simulink model "nao_linear"  (R2025a)
settings: Solver=VariableStepAuto  StartTime=0.0  StopTime=50.0  RelTol=1e-3
values from neighbouring files (symbols this model uses):
  b = 0.010681    [equations_aeropendulum.m]
  den = [1, b/J, (m*g/J) * L1 * cos(theta)]    [equations_aeropendulum.m]
  g = 9.81    [equations_aeropendulum.m]
  J = 0.020218    [equations_aeropendulum.m]
  K = 0.000166    [equations_aeropendulum.m]
  L1 = 0.177    [equations_aeropendulum.m]
  L2 = 0.45    [equations_aeropendulum.m]
  m = 0.218    [equations_aeropendulum.m]
  num = [K * L2 * 2 * pwm / J]    [equations_aeropendulum.m]
  pwm = 89    [equations_aeropendulum.m]
  theta = 90    [equations_aeropendulum.m]
libraries: slpidlib x1
settings Model: Creator=edutera  LastModifiedBy=edutera

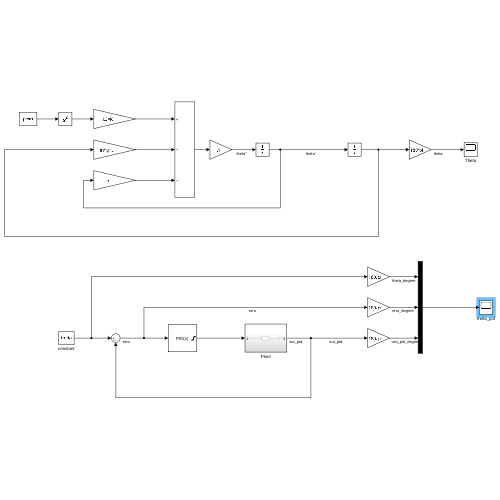
[thumbnail: Simulink's stored preview of the top-level diagram]
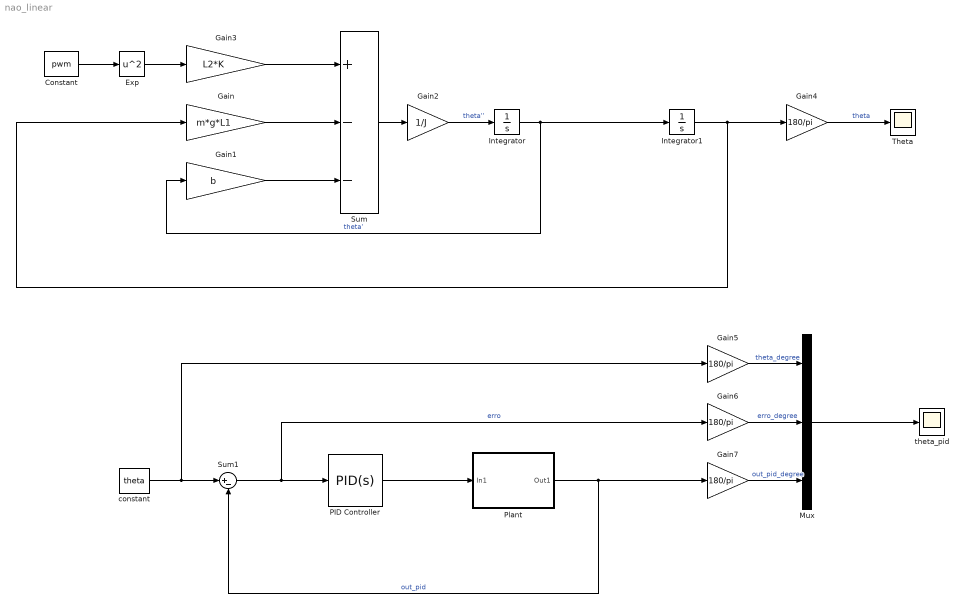
== system nao_linear ==
  Constant : Constant  Value=pwm
  Exp : Math  Operator=square
  Gain : Gain  Gain=m*g*L1
  Gain1 : Gain  Gain=b
  Gain2 : Gain  Gain=1/J
  Gain3 : Gain  Gain=L2*K
  Gain{4..7} (4 alike) : Gain  Gain=180/pi
  Integrator : Integrator
  Integrator1 : Integrator
  Mux : Mux  Inputs=3
  PID Controller : slpidlib/PID Controller  Controller=PID  Form=Parallel  TimeDomain=Continuous-time  UseExternalTs=off  SampleTime=-1  IntegratorMethod=Forward Euler  FilterMethod=Forward Euler  ControllerParametersSource=internal  P=0.5  I=0.06  UseKiTs=off  D=0.9  UseExternalDerivativeSource=off  N=100  UseFilter=on  TunerSelectOption=Transfer Function Based (PID Tuner App)  InitialConditionSource=internal  InitialConditionForIntegrator=0  InitialConditionForFilter=0  DifferentiatorICPrevScaledInput=0  ExternalReset=none  TrackingMode=off  Kt=1  LimitOutput=on  SatLimitsSource=internal  UpperSaturationLimit=255  LowerSaturationLimit=0  LinearizeAsGain=on  AntiWindupMode=clamping  Kb=1  LimitIntegrator=off  UpperIntegratorSaturationLimit=inf  LowerIntegratorSaturationLimit=-inf  POutMin=[]  POutMax=[]  IOutMin=[]  IOutMax=[]  DOutMin=[]  DOutMax=[]  NOutMin=[]  NOutMax=[]  SumOutMin=[]  SumOutMax=[]  SaturationOutMin=[]  SaturationOutMax=[]  PParamMin=[]  PParamMax=[]  IParamMin=[]  IParamMax=[]  DParamMin=[]  DParamMax=[]  NParamMin=[]  NParamMax=[]  KbParamMin=[]  KbParamMax=[]  KtParamMin=[]  KtParamMax=[]  KbOutMin=[]  KbOutMax=[]  KtOutMin=[]  KtOutMax=[]  IntegratorOutMin=[]  IntegratorOutMax=[]  FilterOutMin=[]  FilterOutMax=[]  SumI1OutMin=[]  SumI1OutMax=[]  SumI2OutMin=[]  SumI2OutMax=[]  SumI3OutMin=[]  SumI3OutMax=[]  SumI4OutMin=[]  SumI4OutMax=[]  SumDOutMin=[]  SumDOutMax=[]  DifferentiatorOutMin=[]  DifferentiatorOutMax=[]  FilterDiffOutCoefMin=[]  FilterDiffOutCoefMax=[]  ReciprocalOutMin=[]  ReciprocalOutMax=[]  SumDenOutMin=[]  SumDenOutMax=[]  SumNumOutMin=[]  SumNumOutMax=[]  DivideOutMin=[]  DivideOutMax=[]  UdiffTsProdOutMin=[]  UdiffTsProdOutMax=[]  NTsProdOutMin=[]  NTsProdOutMax=[]  UintegralTsProdOutMin=[]  UintegralTsProdOutMax=[]  UngainTsProdOutMin=[]  UngainTsProdOutMax=[]  ClampingZeroOutDataTypeStr=Inherit: Inherit via back propagation  ClampingZeroOutMin=[]  ClampingZeroOutMax=[]  FilterDenConstantOutDataTypeStr=Inherit: Inherit via back propagation  FilterDenConstantOutMin=[]  FilterDenConstantOutMax=[]  PCopyOutDataTypeStr=Inherit: Inherit via back propagation  PCopyOutMin=[]  PCopyOutMax=[]  NCopyOutDataTypeStr=Inherit: Inherit via back propagation  NCopyOutMin=[]  NCopyOutMax=[]  IntegratorContinuousStateAttributes=''  IntegratorStateMustResolveToSignalObject=off  IntegratorRTWStateStorageClass=Auto  FilterContinuousStateAttributes=''  FilterStateMustResolveToSignalObject=off  FilterRTWStateStorageClass=Auto  ParallelPVariant=InternalParameters  IdealPVariant=Disabled  IVariant=InternalParameters  DVariant=InternalParameters  IntegratorVariant=Continuous  SatVariant=Enabled  AWVariant=ContClampingParallel  PCopyVariant=Disabled  TRVariant=Disabled  FdbkBlocksVariant=Forward  IdealPFdbkVariant=Disabled  SatFdbkVariant=Disabled  DerivativeFilterVariant=ContFilter  NVariant=InternalParameters  NCopyVariant=Disabled  FilterICVariant=InternalICsFilter  IntegratorICVariant=InternalICs  ExternalResetVariant=Disabled  TRSumVariant=Passthrough  SumFdbkVariant=Disabled  SumVariant=Sum_PID  TsampFilterVariant=InternalTs  TsampNgainVariant=Passthrough  TsampIntegralVariant=Disabled_SignalSpec  ExternalSaturationOutDataTypeStr=Inherit: Same as second input  DerivativeSourceVariant=ErrorSignal  PreIntVariant=InternalPreInt
  Plant : Subsystem
  Sum : Sum  Inputs=+--
  Sum1 : Sum  Inputs=|+-
  Theta : Scope
      settings: ActiveDisplayYMinimum=-20.340273426059316  ActiveDisplayYMaximum=183.06246083453388
  constant : Constant  Value=theta
  theta_pid : Scope
      settings: ActiveDisplayYMinimum=-73.196244337252011  ActiveDisplayYMaximum=163.19624433725204
  wires:
  Gain/1 -> Sum/2
  Gain1/1 -> Sum/3
  Integrator/1 -> Gain1/1, Integrator1/1  "theta'"
  Sum/1 -> Gain2/1
  Gain2/1 -> Integrator/1  "theta''"
  Gain3/1 -> Sum/1
  Gain4/1 -> Theta/1  "theta"
  Integrator1/1 -> Gain/1, Gain4/1
  Constant/1 -> Exp/1
  Exp/1 -> Gain3/1
  PID Controller/1 -> Plant/1(In1)
  Plant/1(Out1) -> Gain7/1, Sum1/2  "out_pid"
  Sum1/1 -> Gain6/1, PID Controller/1  "erro"
  Mux/1 -> theta_pid/1
  Gain5/1 -> Mux/1  "theta_degree"
  Gain6/1 -> Mux/2  "erro_degree"
  Gain7/1 -> Mux/3  "out_pid_degree"
  constant/1 -> Gain5/1, Sum1/1

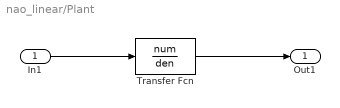
== system nao_linear/Plant ==
  In1 : Inport
  Transfer Fcn : TransferFcn  Numerator=num  Denominator=den
  Out1 : Outport
  wires:
  Transfer Fcn/1 -> Out1/1
  In1/1 -> Transfer Fcn/1
